simulink model "eCS_Algo_Simulation_2015b"  (R2015b)
settings: Solver=ode1  StartTime=0.0  StopTime=3  FixedStep=1/80000  RelTol=1e-3
PreLoadFcn:
  | if exist('tl_preloadfcn','file'), tl_preloadfcn(gcs,402); end
PostLoadFcn:
  | , if any(exist('dsrtsu_mdlpostloadfcn', 'file') == [2, 3, 6]), try dsrtsu_mdlpostloadfcn('Execute', bdroot); catch fprintf('Error in PostLoadFcn (dsrtsu_mdlpostloadfcn) for model "%s":\n %s\n', bdroot, lasterr); end, end,
  | if exist('tl_postloadfcn','file'), tl_postloadfcn(gcs,402); end
InitFcn:
  | Omegan=1.3024e+03;
  | xi=0.9; %0.48
  | K=0.1931;
  | K1=0.0198;
  | TauLocked=0.00255;
  | TauUnLocked=0.0042;
  | Kp=1/(2*K1);
  | Ki=Kp/((TauLocked+TauUnLocked)/2);
  | if exist('tlds_init','file'), tlds_init(gcs); end
StartFcn:
  | if exist('tlds_start','file'), tlds_start(gcs); end
StopFcn:
  | if exist('tlds_stop','file'), tlds_stop(gcs); end
model workspace (MAT data in the model file):
  au8PrevExecProfile = [0 0 0 0 0 0]
values from neighbouring files (symbols this model uses):
  AccSensor = 5    [Parameter_eCS_Algo.m]
  AlgoType = 0    [Parameter_eCS_Algo.m]
  Cxy = 1*0.017    (= 0.017)    [Acc_Init_SelV1.m]
  Cxz = 1*0.017    (= 0.017)    [Acc_Init_SelV1.m]
  Cyx = 1*0.017    (= 0.017)    [Acc_Init_SelV1.m]
  Cyz = 1*0.017    (= 0.017)    [Acc_Init_SelV1.m]
  Czx = 1*0.017    (= 0.017)    [Acc_Init_SelV1.m]
  Czy = 1*0.017    (= 0.017)    [Acc_Init_SelV1.m]
  Forced_Oscillation = 0    [Parameter_eCS_Algo.m]    (also in run_Rotation_sim.m = run)
  FreqTemperature = 10    [Acc_Init_SelV1.m]
  MaxSensorOffset = 0.3    [Acc_Init_SelV1.m]
  Mean_x_noise = 4e-3    (= 0.004)    [Acc_Init_SelV1.m]
  Mean_y_noise = 4e-3    (= 0.004)    [Acc_Init_SelV1.m]
  Mean_z_noise = 4e-3    (= 0.004)    [Acc_Init_SelV1.m]
  ODR = 8000    [Acc_Init_SelV1.m]
  offsetcorrection_on_off = 0    [Parameter_eCS_Algo.m]
  phi_pulse_rotation = 0    [Parameter_eCS_Algo.m]    (also in run_Rotation_sim.m = angle)
  pulsetype = 2    [Parameter_eCS_Algo.m]    (also in run_simulation.m = j; run_simulation_ActiveX.m = j)
  Range = 4    [Acc_Init_SelV1.m]
  sensitivity_optimisation = 0    [Parameter_eCS_Algo.m]
  TempBias = 0    [Acc_Init_SelV1.m]
  TemperatureAmp = 0    [Acc_Init_SelV1.m]
  Var_x_noise = 1.84e-9    (= 1.84e-09)    [Acc_Init_SelV1.m]
  Var_y_noise = 2.025e-09    [Acc_Init_SelV1.m]
  Var_z_noise = 1.374e-09    [Acc_Init_SelV1.m]
  w_x = 2*pi*F_x    (= 376.991118431)    [Acc_Init_SelV1.m]
  w_y = 2*pi*F_y    (= 376.991118431)    [Acc_Init_SelV1.m]
  w_z = 2*pi*F_z    (= 376.991118431)    [Acc_Init_SelV1.m]
  x_max_temp_drift = 0.061    [Acc_Init_SelV1.m]
  x_offset_enable = 0    [Acc_Init_SelV1.m]
  x_run_to_run_drift = 0.0    (= 0)    [Acc_Init_SelV1.m]
  x_temp_co_drift = 0.000    (= 0)    [Acc_Init_SelV1.m]
  Xi_x = 0.7    [Acc_Init_SelV1.m]
  Xi_y = 0.7    [Acc_Init_SelV1.m]
  Xi_z = 0.7    [Acc_Init_SelV1.m]
  y_max_temp_drift = 0.061    [Acc_Init_SelV1.m]
  y_offset_enable = 0    [Acc_Init_SelV1.m]
  y_run_to_run_drift = 0.0    (= 0)    [Acc_Init_SelV1.m]
  y_temp_co_drift = 0.000    (= 0)    [Acc_Init_SelV1.m]
  z_max_temp_drift = 0.13    [Acc_Init_SelV1.m]
  z_offset_enable = 0    [Acc_Init_SelV1.m]
  z_run_to_run_drift = 0.0    (= 0)    [Acc_Init_SelV1.m]
  z_temp_co_drift = 0.000    (= 0)    [Acc_Init_SelV1.m]
undefined symbols (not defined in the file or in its folder): controller_sample_rate, ddv, DiscIntNeverNeededParam, gmw_roada_x__m_s__, gmw_roada_y__m_s__, gmw_roadtime_2kHz, KSF_50_a_x, KSF_50_a_y, KSF_50_time, KSG_30_a_x, KSG_30_a_y, KSG_30_time, Meldorf_HindenburgstraAcceleration_x__m_s_2_, Meldorf_HindenburgstraAcceleration_y__m_s_2_, Meldorf_HindenburgstraAcceleration_z__m_s_2_, Meldorf_HindenburgstraTime__s_, pulse_FF27, pulse_MPDB, pulse_ODB40, pulse_ODB64, pulse_USNCAP, pulsetime_FF27, pulsetime_MPDB, pulsetime_ODB40, pulsetime_ODB64, pulsetime_USNCAP, Rauasphalt_60_a_x, Rauasphalt_60_a_y, Rauasphalt_60_time, sigbuilder_block, VW_416_2kHza_x_2kHz, VW_416_2kHza_y_2kHz, VW_416_2kHztime_2kHz
libraries: simulink x29, tllib x23, tl_autosar_lib x15, simulink_extras x7, LIB_TF_G_111 x2, LIB_TF_G_12_StepControl x2, LIB_TF_G_112 x1, dspsigops x1
(part 10 of 13)

== system eCS_Algo_Simulation_2015b/SAD/Subsystem/SAD/SAD/SAD_runMainFunction/SAD mainfunction/Check for following profile ==
  profile : Inport
  PrevStepIdx : Inport  Port=2
  stProfileCfg : Inport  Port=3
  Action Port : ActionPort  ActionType=then
  Check for following profile : Subsystem  TreatAsAtomicUnit=on
  Constant8 : Constant  Value=ddv('SAD/Macros/Profiles/KU8_NO_PROFILE')  mask(TL_Constant){data={'output',{'variable','SAD/Macros/Profiles/KU8_NO_PROFILE'},'date',738430.41690531245}}
      settings: CopyFcn=if exist('tl_reset_reviewflag','file')==2,tl_reset_reviewflag(gcbh);end  DeleteFcn=if exist('delete_tlblock','file')==2,delete_tlblock(gcbh);end  NameChangeFcn=if exist('rename_tlblock','file')==2,rename_tlblock(gcbh);end  OpenFcn=if exist('tl_open_blockdlg','file')==2,tl_open_blockdlg(gcbh);else,open_system(gcbh,'parameter');end
      mask Help: eval(['if exist(''tl_online_help'',''file'') == 2, tl_online_help(''Topic'',''TL_Constant''),else, web([''jar:file:///'',matlabroot,''/help/toolbox/simulink/help.jar!/slref/' lower(get_param(gcbh,'Blocktype')) '.html''], ''-helpbrowser''),end'])
      mask Display: plot([-0.1, 1.05, NaN, -0.1, 1.05],[.01, .01, NaN, .99, .99]);
  If : If  IfExpression=u1
  Keep current one : Subsystem  TreatAsAtomicUnit=on
  Merge : Merge  mask(TL_Merge){data={'date',738430.416905544}}
      settings: CopyFcn=if exist('tl_reset_reviewflag') == 2, tl_reset_reviewflag(gcbh); end  DeleteFcn=if exist('delete_tlblock','file')==2,delete_tlblock(gcbh);end  NameChangeFcn=if exist('rename_tlblock','file')==2,rename_tlblock(gcbh);end  OpenFcn=if exist('tl_open_blockdlg','file')==2,tl_open_blockdlg(gcbh);else,open_system(gcbh,'parameter');end
      mask Help: eval(['if exist(''tl_online_help'',''file'') == 2, tl_online_help(''Topic'',''TL_Merge''),else, web([''jar:file:///'',matlabroot,''/help/toolbox/simulink/help.jar!/slref/' lower(get_param(gcbh,'Blocktype')) '.html''], ''-helpbrowser''),end'])
      mask Display: plot([-0.1, 1.05, NaN, -0.1, 1.05],[.01, .01, NaN, .99, .99]);
  Relational Operator2 : RelationalOperator  Operator=~=  OutDataTypeStr=boolean  mask(TL_RelationalOperator){data={'date',738430.41690565972}}
      settings: DeleteFcn=if exist('delete_tlblock','file')==2,delete_tlblock(gcbh);end  NameChangeFcn=if exist('rename_tlblock','file')==2,rename_tlblock(gcbh);end  OpenFcn=if exist('tl_open_blockdlg','file')==2,tl_open_blockdlg(gcbh);else,open_system(gcbh,'parameter');end
      mask Help: eval(['if exist(''tl_online_help'',''file'') == 2, tl_online_help(''Topic'',''TL_RelationalOperator''),else, web([''jar:file:///'',matlabroot,''/help/toolbox/simulink/help.jar!/slref/' lower(get_param(gcbh,'Blocktype')) '.html''], ''-helpbrowser''),end'])
      mask Display: plot([-0.1, 1.05, NaN, -0.1, 1.05],[.01, .01, NaN, .99, .99]);
  selectedProfile : Outport
  wires:
  If/1 -> Check for following profile/Action
  Constant8/1 -> Relational Operator2/2
  Relational Operator2/1 -> If/1
  If/2 -> Keep current one/Action
  Check for following profile/1(Out1) -> Merge/1
  Keep current one/1(Out1) -> Merge/2
  Merge/1 -> selectedProfile/1
  PrevStepIdx/1 -> Check for following profile/1(PrevStepIdx)
  profile/1 -> Check for following profile/3(SelectedProfile), Keep current one/1(profile), Relational Operator2/1
  stProfileCfg/1 -> Check for following profile/2(stProfileCfg)

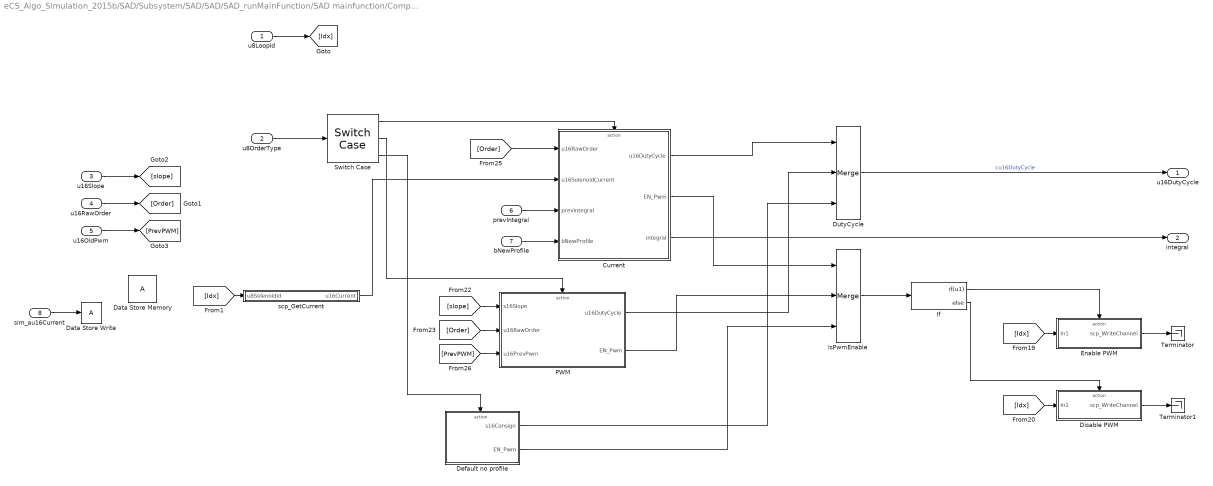
== system eCS_Algo_Simulation_2015b/SAD/Subsystem/SAD/SAD/SAD_runMainFunction/SAD mainfunction/ComputeDutyCycle ==
  u8LoopId : Inport
  u8OrderType : Inport  Port=2
  u16Slope : Inport  Port=3
  u16RawOrder : Inport  Port=4
  u16OldPwm : Inport  Port=5
  prevIntegral : Inport  Port=6
  bNewProfile : Inport  Port=7
  sim_au16Current : Inport  Port=8
  Current : Subsystem  TreatAsAtomicUnit=on
  Data Store Memory : DataStoreMemory  ReadBeforeWriteMsg=warning  WriteAfterWriteMsg=warning  WriteAfterReadMsg=warning  InitialValue=[0 0 0 0 0 0]  mask(TL_DataStoreMemory){data={'output',{'type','UInt16'},'date',738433.70621954859}}
      settings: CopyFcn=if exist('tl_reset_reviewflag') == 2, tl_reset_reviewflag(gcbh); end  DeleteFcn=if exist('delete_tlblock','file')==2,delete_tlblock(gcbh);end  NameChangeFcn=if exist('rename_tlblock','file')==2,rename_tlblock(gcbh);end  OpenFcn=if exist('tl_open_blockdlg','file')==2,tl_open_blockdlg(gcbh);else,open_system(gcbh,'parameter');end
      mask Help: eval(['if exist(''tl_online_help'',''file'') == 2, tl_online_help(''Topic'',''TL_DataStoreMemory''),else, web([''jar:file:///'',matlabroot,''/help/toolbox/simulink/help.jar!/slref/' lower(get_param(gcbh,'Blocktype')) '.html''], ''-helpbrowser''),end'])
      mask Display:
      | plot([-0.1, 1.05, NaN, -0.1, 1.05],[.01, .01, NaN, .99, .99]);
      | plot([-0.1, 1.05, NaN, -0.1, 1.05],[.01, .01, NaN, .99, .99]);
  Data Store Write : DataStoreWrite  mask(TL_DataStoreWrite){data={'date',738433.42894126161}}
      settings: DeleteFcn=if exist('delete_tlblock','file')==2,delete_tlblock(gcbh);end  NameChangeFcn=if exist('rename_tlblock','file')==2,rename_tlblock(gcbh);end  OpenFcn=if exist('tl_open_blockdlg','file')==2,tl_open_blockdlg(gcbh);else,open_system(gcbh,'parameter');end
      mask Help: eval(['if exist(''tl_online_help'',''file'') == 2, tl_online_help(''Topic'',''TL_DataStoreWrite''),else, web([''jar:file:///'',matlabroot,''/help/toolbox/simulink/help.jar!/slref/' lower(get_param(gcbh,'Blocktype')) '.html''], ''-helpbrowser''),end'])
      mask Display: plot([-0.1, 1.05, NaN, -0.1, 1.05],[.01, .01, NaN, .99, .99]);
  Default no profile : Subsystem  TreatAsAtomicUnit=on
  Disable PWM : Subsystem  TreatAsAtomicUnit=on
  DutyCycle : Merge  Inputs=3  mask(TL_Merge){data={'date',738430.41690787033}}
      settings: CopyFcn=if exist('tl_reset_reviewflag') == 2, tl_reset_reviewflag(gcbh); end  DeleteFcn=if exist('delete_tlblock','file')==2,delete_tlblock(gcbh);end  NameChangeFcn=if exist('rename_tlblock','file')==2,rename_tlblock(gcbh);end  OpenFcn=if exist('tl_open_blockdlg','file')==2,tl_open_blockdlg(gcbh);else,open_system(gcbh,'parameter');end
      mask Help: eval(['if exist(''tl_online_help'',''file'') == 2, tl_online_help(''Topic'',''TL_Merge''),else, web([''jar:file:///'',matlabroot,''/help/toolbox/simulink/help.jar!/slref/' lower(get_param(gcbh,'Blocktype')) '.html''], ''-helpbrowser''),end'])
      mask Display: plot([-0.1, 1.05, NaN, -0.1, 1.05],[.01, .01, NaN, .99, .99]);
  Enable PWM : Subsystem  TreatAsAtomicUnit=on
  If : If  IfExpression=u1
  IsPwmEnable : Merge  Inputs=3  mask(TL_Merge){data={'date',738430.41690775461}}
      settings: CopyFcn=if exist('tl_reset_reviewflag') == 2, tl_reset_reviewflag(gcbh); end  DeleteFcn=if exist('delete_tlblock','file')==2,delete_tlblock(gcbh);end  NameChangeFcn=if exist('rename_tlblock','file')==2,rename_tlblock(gcbh);end  OpenFcn=if exist('tl_open_blockdlg','file')==2,tl_open_blockdlg(gcbh);else,open_system(gcbh,'parameter');end
      mask Help: eval(['if exist(''tl_online_help'',''file'') == 2, tl_online_help(''Topic'',''TL_Merge''),else, web([''jar:file:///'',matlabroot,''/help/toolbox/simulink/help.jar!/slref/' lower(get_param(gcbh,'Blocktype')) '.html''], ''-helpbrowser''),end'])
      mask Display: plot([-0.1, 1.05, NaN, -0.1, 1.05],[.01, .01, NaN, .99, .99]);
  PWM : Subsystem  TreatAsAtomicUnit=on
  Switch Case : SwitchCase  CaseConditions={1,2}
  Terminator : Terminator
  Terminator1 : Terminator
  scp_GetCurrent : Subsystem  TreatAsAtomicUnit=on
  u16DutyCycle : Outport
  integral : Outport  Port=2
  wires:
  u8OrderType/1 -> Switch Case/1
  Switch Case/3 -> Default no profile/Action
  Default no profile/2(EN_Pwm) -> IsPwmEnable/3
  If/1 -> Enable PWM/Action
  Default no profile/1(s16Consign) -> DutyCycle/3
  [Idx] -> Disable PWM/1(In1)
  Disable PWM/1(scp_WriteChannel) -> Terminator1/1
  [PrevPWM] -> PWM/3(u16PrevPwm)
  [Order] -> Current/1(u16RawOrder)
  [Order] -> PWM/2(u16RawOrder)
  Enable PWM/1(scp_WriteChannel) -> Terminator/1
  [Idx] -> Enable PWM/1(In1)
  If/2 -> Disable PWM/Action
  [slope] -> PWM/1(s16Slope)
  DutyCycle/1 -> u16DutyCycle/1  "cu16DutyCycle"
  Switch Case/1 -> Current/Action
  Switch Case/2 -> PWM/Action
  u8LoopId/1 -> [Idx]
  u16RawOrder/1 -> [Order]
  u16Slope/1 -> [slope]
  u16OldPwm/1 -> [PrevPWM]
  IsPwmEnable/1 -> If/1
  [Idx] -> scp_GetCurrent/1(u8SolenoidId)
  scp_GetCurrent/1(u16Current) -> Current/2(u16SolenoidCurrent)
  Current/3(integral) -> integral/1
  prevIntegral/1 -> Current/3(prevIntegral)
  bNewProfile/1 -> Current/4(bNewProfile)
  sim_au16Current/1 -> Data Store Write/1
  Current/2(EN_Pwm) -> IsPwmEnable/1
  PWM/2(EN_Pwm) -> IsPwmEnable/2
  Current/1(u16DutyCycle) -> DutyCycle/1
  PWM/1(u16DutyCycle) -> DutyCycle/2

== system eCS_Algo_Simulation_2015b/SAD/Subsystem/SAD/SAD/SAD_runMainFunction/SAD mainfunction/Keep current profile ==
  PrevProfile : Inport
  Action Port : ActionPort  ActionType=else
  SelectedProfile : Outport
  wires:
  PrevProfile/1 -> SelectedProfile/1

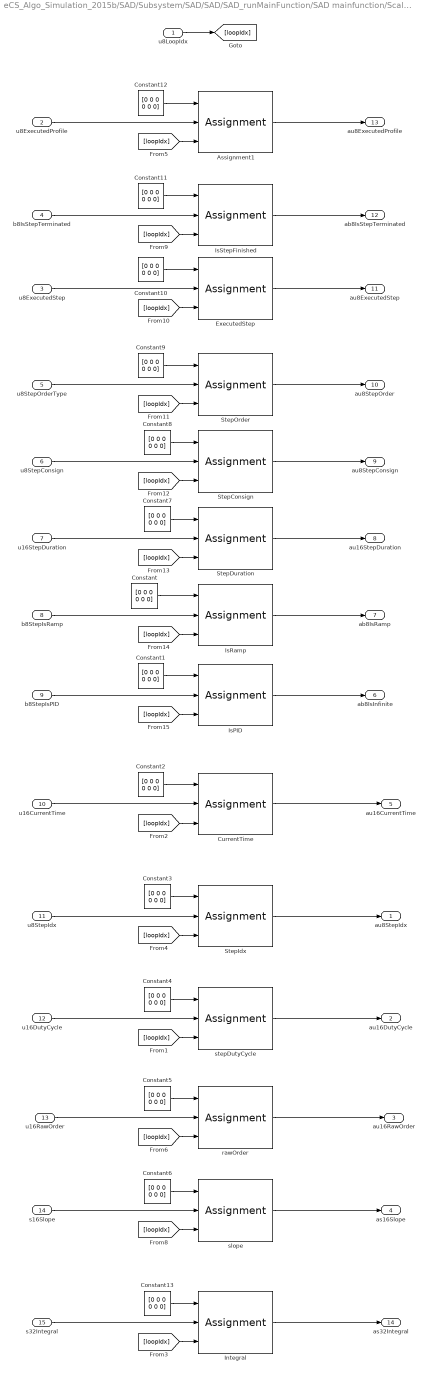
== system eCS_Algo_Simulation_2015b/SAD/Subsystem/SAD/SAD/SAD_runMainFunction/SAD mainfunction/ScalarToVector ==
  u8LoopIdx : Inport
  u8ExecutedProfile : Inport  Port=2
  u8ExecutedStep : Inport  Port=3
  b8IsStepTerminated : Inport  Port=4
  u8StepOrderType : Inport  Port=5
  u8StepConsign : Inport  Port=6
  u16StepDuration : Inport  Port=7
  b8StepIsRamp : Inport  Port=8
  b8StepIsPID : Inport  Port=9
  u16CurrentTime : Inport  Port=10
  u8StepIdx : Inport  Port=11
  u16DutyCycle : Inport  Port=12
  u16RawOrder : Inport  Port=13
  s16Slope : Inport  Port=14
  s32Integral : Inport  Port=15
  Assignment1 : Assignment  IndexMode=Zero-based  IndexOptions=Index vector (port)  Indices=1  OutputSizes=1  mask(TL_Assignment){data={'insideiteratedsystem',logical(1),'omitinitializations',1,'output',{'variable','SAD/Vars/Profiles/au8ExecProfile','inheritscaling',0},'date',738430.41691026615}}
      settings: CopyFcn=if exist('tl_reset_reviewflag') == 2, tl_reset_reviewflag(gcbh); end  DeleteFcn=if exist('delete_tlblock','file')==2,delete_tlblock(gcbh);end  NameChangeFcn=if exist('rename_tlblock','file')==2,rename_tlblock(gcbh);end  OpenFcn=if exist('tl_open_blockdlg','file')==2,tl_open_blockdlg(gcbh);else,open_system(gcbh,'parameter');end
      mask Help: eval(['if exist(''tl_online_help'',''file'') == 2, tl_online_help(''Topic'',''TL_Assignment''),else, web([''jar:file:///'',matlabroot,''/help/toolbox/simulink/help.jar!/slref/' lower(get_param(gcbh,'Blocktype')) '.html''], ''-helpbrowser''),end'])
      mask Display: plot([-0.1, 1.05, NaN, -0.1, 1.05],[.01, .01, NaN, .99, .99]);
  Constant : Constant  Value=[0 0 0 0 0 0]  mask(TL_Constant){data={'date',738430.41691038199}}
      settings: CopyFcn=if exist('tl_reset_reviewflag') == 2, tl_reset_reviewflag(gcbh); end  DeleteFcn=if exist('delete_tlblock','file')==2,delete_tlblock(gcbh);end  NameChangeFcn=if exist('rename_tlblock','file')==2,rename_tlblock(gcbh);end  OpenFcn=if exist('tl_open_blockdlg','file')==2,tl_open_blockdlg(gcbh);else,open_system(gcbh,'parameter');end
      mask Help: eval(['if exist(''tl_online_help'',''file'') == 2, tl_online_help(''Topic'',''TL_Constant''),else, web([''jar:file:///'',matlabroot,''/help/toolbox/simulink/help.jar!/slref/' lower(get_param(gcbh,'Blocktype')) '.html''], ''-helpbrowser''),end'])
      mask Display: plot([-0.1, 1.05, NaN, -0.1, 1.05],[.01, .01, NaN, .99, .99]);
  Constant1 : Constant  Value=[0 0 0 0 0 0]  mask(TL_Constant){data={'date',738430.4169104977}}
      settings: CopyFcn=if exist('tl_reset_reviewflag') == 2, tl_reset_reviewflag(gcbh); end  DeleteFcn=if exist('delete_tlblock','file')==2,delete_tlblock(gcbh);end  NameChangeFcn=if exist('rename_tlblock','file')==2,rename_tlblock(gcbh);end  OpenFcn=if exist('tl_open_blockdlg','file')==2,tl_open_blockdlg(gcbh);else,open_system(gcbh,'parameter');end
      mask Help: eval(['if exist(''tl_online_help'',''file'') == 2, tl_online_help(''Topic'',''TL_Constant''),else, web([''jar:file:///'',matlabroot,''/help/toolbox/simulink/help.jar!/slref/' lower(get_param(gcbh,'Blocktype')) '.html''], ''-helpbrowser''),end'])
      mask Display: plot([-0.1, 1.05, NaN, -0.1, 1.05],[.01, .01, NaN, .99, .99]);
  Constant10 : Constant  Value=[0 0 0 0 0 0]  mask(TL_Constant){data={'date',738430.41691072914}}
      settings: CopyFcn=if exist('tl_reset_reviewflag') == 2, tl_reset_reviewflag(gcbh); end  DeleteFcn=if exist('delete_tlblock','file')==2,delete_tlblock(gcbh);end  NameChangeFcn=if exist('rename_tlblock','file')==2,rename_tlblock(gcbh);end  OpenFcn=if exist('tl_open_blockdlg','file')==2,tl_open_blockdlg(gcbh);else,open_system(gcbh,'parameter');end
      mask Help: eval(['if exist(''tl_online_help'',''file'') == 2, tl_online_help(''Topic'',''TL_Constant''),else, web([''jar:file:///'',matlabroot,''/help/toolbox/simulink/help.jar!/slref/' lower(get_param(gcbh,'Blocktype')) '.html''], ''-helpbrowser''),end'])
      mask Display: plot([-0.1, 1.05, NaN, -0.1, 1.05],[.01, .01, NaN, .99, .99]);
  Constant11 : Constant  Value=[0 0 0 0 0 0]  mask(TL_Constant){data={'date',738430.4169108565}}
      settings: CopyFcn=if exist('tl_reset_reviewflag') == 2, tl_reset_reviewflag(gcbh); end  DeleteFcn=if exist('delete_tlblock','file')==2,delete_tlblock(gcbh);end  NameChangeFcn=if exist('rename_tlblock','file')==2,rename_tlblock(gcbh);end  OpenFcn=if exist('tl_open_blockdlg','file')==2,tl_open_blockdlg(gcbh);else,open_system(gcbh,'parameter');end
      mask Help: eval(['if exist(''tl_online_help'',''file'') == 2, tl_online_help(''Topic'',''TL_Constant''),else, web([''jar:file:///'',matlabroot,''/help/toolbox/simulink/help.jar!/slref/' lower(get_param(gcbh,'Blocktype')) '.html''], ''-helpbrowser''),end'])
      mask Display: plot([-0.1, 1.05, NaN, -0.1, 1.05],[.01, .01, NaN, .99, .99]);
  Constant12 : Constant  Value=[0 0 0 0 0 0]  mask(TL_Constant){data={'date',738430.41691097221}}
      settings: CopyFcn=if exist('tl_reset_reviewflag') == 2, tl_reset_reviewflag(gcbh); end  DeleteFcn=if exist('delete_tlblock','file')==2,delete_tlblock(gcbh);end  NameChangeFcn=if exist('rename_tlblock','file')==2,rename_tlblock(gcbh);end  OpenFcn=if exist('tl_open_blockdlg','file')==2,tl_open_blockdlg(gcbh);else,open_system(gcbh,'parameter');end
      mask Help: eval(['if exist(''tl_online_help'',''file'') == 2, tl_online_help(''Topic'',''TL_Constant''),else, web([''jar:file:///'',matlabroot,''/help/toolbox/simulink/help.jar!/slref/' lower(get_param(gcbh,'Blocktype')) '.html''], ''-helpbrowser''),end'])
      mask Display: plot([-0.1, 1.05, NaN, -0.1, 1.05],[.01, .01, NaN, .99, .99]);
  Constant13 : Constant  Value=[0 0 0 0 0 0]  mask(TL_Constant){data={'date',738430.41691166663}}
      settings: CopyFcn=if exist('tl_reset_reviewflag') == 2, tl_reset_reviewflag(gcbh); end  DeleteFcn=if exist('delete_tlblock','file')==2,delete_tlblock(gcbh);end  NameChangeFcn=if exist('rename_tlblock','file')==2,rename_tlblock(gcbh);end  OpenFcn=if exist('tl_open_blockdlg','file')==2,tl_open_blockdlg(gcbh);else,open_system(gcbh,'parameter');end
      mask Help: eval(['if exist(''tl_online_help'',''file'') == 2, tl_online_help(''Topic'',''TL_Constant''),else, web([''jar:file:///'',matlabroot,''/help/toolbox/simulink/help.jar!/slref/' lower(get_param(gcbh,'Blocktype')) '.html''], ''-helpbrowser''),end'])
      mask Display: plot([-0.1, 1.05, NaN, -0.1, 1.05],[.01, .01, NaN, .99, .99]);
  Constant2 : Constant  Value=[0 0 0 0 0 0]  mask(TL_Constant){data={'date',738430.41691108793}}
      settings: CopyFcn=if exist('tl_reset_reviewflag') == 2, tl_reset_reviewflag(gcbh); end  DeleteFcn=if exist('delete_tlblock','file')==2,delete_tlblock(gcbh);end  NameChangeFcn=if exist('rename_tlblock','file')==2,rename_tlblock(gcbh);end  OpenFcn=if exist('tl_open_blockdlg','file')==2,tl_open_blockdlg(gcbh);else,open_system(gcbh,'parameter');end
      mask Help: eval(['if exist(''tl_online_help'',''file'') == 2, tl_online_help(''Topic'',''TL_Constant''),else, web([''jar:file:///'',matlabroot,''/help/toolbox/simulink/help.jar!/slref/' lower(get_param(gcbh,'Blocktype')) '.html''], ''-helpbrowser''),end'])
      mask Display: plot([-0.1, 1.05, NaN, -0.1, 1.05],[.01, .01, NaN, .99, .99]);
  Constant3 : Constant  Value=[0 0 0 0 0 0]  mask(TL_Constant){data={'date',738430.41691120365}}
      settings: CopyFcn=if exist('tl_reset_reviewflag') == 2, tl_reset_reviewflag(gcbh); end  DeleteFcn=if exist('delete_tlblock','file')==2,delete_tlblock(gcbh);end  NameChangeFcn=if exist('rename_tlblock','file')==2,rename_tlblock(gcbh);end  OpenFcn=if exist('tl_open_blockdlg','file')==2,tl_open_blockdlg(gcbh);else,open_system(gcbh,'parameter');end
      mask Help: eval(['if exist(''tl_online_help'',''file'') == 2, tl_online_help(''Topic'',''TL_Constant''),else, web([''jar:file:///'',matlabroot,''/help/toolbox/simulink/help.jar!/slref/' lower(get_param(gcbh,'Blocktype')) '.html''], ''-helpbrowser''),end'])
      mask Display: plot([-0.1, 1.05, NaN, -0.1, 1.05],[.01, .01, NaN, .99, .99]);
  Constant4 : Constant  Value=[0 0 0 0 0 0]  mask(TL_Constant){data={'date',738430.41691131948}}
      settings: CopyFcn=if exist('tl_reset_reviewflag') == 2, tl_reset_reviewflag(gcbh); end  DeleteFcn=if exist('delete_tlblock','file')==2,delete_tlblock(gcbh);end  NameChangeFcn=if exist('rename_tlblock','file')==2,rename_tlblock(gcbh);end  OpenFcn=if exist('tl_open_blockdlg','file')==2,tl_open_blockdlg(gcbh);else,open_system(gcbh,'parameter');end
      mask Help: eval(['if exist(''tl_online_help'',''file'') == 2, tl_online_help(''Topic'',''TL_Constant''),else, web([''jar:file:///'',matlabroot,''/help/toolbox/simulink/help.jar!/slref/' lower(get_param(gcbh,'Blocktype')) '.html''], ''-helpbrowser''),end'])
      mask Display: plot([-0.1, 1.05, NaN, -0.1, 1.05],[.01, .01, NaN, .99, .99]);
  Constant5 : Constant  Value=[0 0 0 0 0 0]  mask(TL_Constant){data={'date',738430.41691155091}}
      settings: CopyFcn=if exist('tl_reset_reviewflag') == 2, tl_reset_reviewflag(gcbh); end  DeleteFcn=if exist('delete_tlblock','file')==2,delete_tlblock(gcbh);end  NameChangeFcn=if exist('rename_tlblock','file')==2,rename_tlblock(gcbh);end  OpenFcn=if exist('tl_open_blockdlg','file')==2,tl_open_blockdlg(gcbh);else,open_system(gcbh,'parameter');end
      mask Help: eval(['if exist(''tl_online_help'',''file'') == 2, tl_online_help(''Topic'',''TL_Constant''),else, web([''jar:file:///'',matlabroot,''/help/toolbox/simulink/help.jar!/slref/' lower(get_param(gcbh,'Blocktype')) '.html''], ''-helpbrowser''),end'])
      mask Display: plot([-0.1, 1.05, NaN, -0.1, 1.05],[.01, .01, NaN, .99, .99]);
  Constant6 : Constant  Value=[0 0 0 0 0 0]  mask(TL_Constant){data={'date',738430.41691166663}}
      settings: CopyFcn=if exist('tl_reset_reviewflag') == 2, tl_reset_reviewflag(gcbh); end  DeleteFcn=if exist('delete_tlblock','file')==2,delete_tlblock(gcbh);end  NameChangeFcn=if exist('rename_tlblock','file')==2,rename_tlblock(gcbh);end  OpenFcn=if exist('tl_open_blockdlg','file')==2,tl_open_blockdlg(gcbh);else,open_system(gcbh,'parameter');end
      mask Help: eval(['if exist(''tl_online_help'',''file'') == 2, tl_online_help(''Topic'',''TL_Constant''),else, web([''jar:file:///'',matlabroot,''/help/toolbox/simulink/help.jar!/slref/' lower(get_param(gcbh,'Blocktype')) '.html''], ''-helpbrowser''),end'])
      mask Display: plot([-0.1, 1.05, NaN, -0.1, 1.05],[.01, .01, NaN, .99, .99]);
  Constant7 : Constant  Value=[0 0 0 0 0 0]  mask(TL_Constant){data={'date',738430.41691178246}}
      settings: CopyFcn=if exist('tl_reset_reviewflag') == 2, tl_reset_reviewflag(gcbh); end  DeleteFcn=if exist('delete_tlblock','file')==2,delete_tlblock(gcbh);end  NameChangeFcn=if exist('rename_tlblock','file')==2,rename_tlblock(gcbh);end  OpenFcn=if exist('tl_open_blockdlg','file')==2,tl_open_blockdlg(gcbh);else,open_system(gcbh,'parameter');end
      mask Help: eval(['if exist(''tl_online_help'',''file'') == 2, tl_online_help(''Topic'',''TL_Constant''),else, web([''jar:file:///'',matlabroot,''/help/toolbox/simulink/help.jar!/slref/' lower(get_param(gcbh,'Blocktype')) '.html''], ''-helpbrowser''),end'])
      mask Display: plot([-0.1, 1.05, NaN, -0.1, 1.05],[.01, .01, NaN, .99, .99]);
  Constant8 : Constant  Value=[0 0 0 0 0 0]  mask(TL_Constant){data={'date',738430.41691189818}}
      settings: CopyFcn=if exist('tl_reset_reviewflag') == 2, tl_reset_reviewflag(gcbh); end  DeleteFcn=if exist('delete_tlblock','file')==2,delete_tlblock(gcbh);end  NameChangeFcn=if exist('rename_tlblock','file')==2,rename_tlblock(gcbh);end  OpenFcn=if exist('tl_open_blockdlg','file')==2,tl_open_blockdlg(gcbh);else,open_system(gcbh,'parameter');end
      mask Help: eval(['if exist(''tl_online_help'',''file'') == 2, tl_online_help(''Topic'',''TL_Constant''),else, web([''jar:file:///'',matlabroot,''/help/toolbox/simulink/help.jar!/slref/' lower(get_param(gcbh,'Blocktype')) '.html''], ''-helpbrowser''),end'])
      mask Display: plot([-0.1, 1.05, NaN, -0.1, 1.05],[.01, .01, NaN, .99, .99]);
  Constant9 : Constant  Value=[0 0 0 0 0 0]  mask(TL_Constant){data={'date',738430.41691199073}}
      settings: CopyFcn=if exist('tl_reset_reviewflag') == 2, tl_reset_reviewflag(gcbh); end  DeleteFcn=if exist('delete_tlblock','file')==2,delete_tlblock(gcbh);end  NameChangeFcn=if exist('rename_tlblock','file')==2,rename_tlblock(gcbh);end  OpenFcn=if exist('tl_open_blockdlg','file')==2,tl_open_blockdlg(gcbh);else,open_system(gcbh,'parameter');end
      mask Help: eval(['if exist(''tl_online_help'',''file'') == 2, tl_online_help(''Topic'',''TL_Constant''),else, web([''jar:file:///'',matlabroot,''/help/toolbox/simulink/help.jar!/slref/' lower(get_param(gcbh,'Blocktype')) '.html''], ''-helpbrowser''),end'])
      mask Display: plot([-0.1, 1.05, NaN, -0.1, 1.05],[.01, .01, NaN, .99, .99]);
  CurrentTime : Assignment  IndexMode=Zero-based  IndexOptions=Index vector (port)  Indices=1  OutputSizes=1  mask(TL_Assignment){data={'insideiteratedsystem',logical(1),'omitinitializations',1,'output',{'variable','SAD/Vars/Steps/au16Time','inheritscaling',0},'date',738430.41691224533}}
      settings: CopyFcn=if exist('tl_reset_reviewflag') == 2, tl_reset_reviewflag(gcbh); end  DeleteFcn=if exist('delete_tlblock','file')==2,delete_tlblock(gcbh);end  NameChangeFcn=if exist('rename_tlblock','file')==2,rename_tlblock(gcbh);end  OpenFcn=if exist('tl_open_blockdlg','file')==2,tl_open_blockdlg(gcbh);else,open_system(gcbh,'parameter');end
      mask Help: eval(['if exist(''tl_online_help'',''file'') == 2, tl_online_help(''Topic'',''TL_Assignment''),else, web([''jar:file:///'',matlabroot,''/help/toolbox/simulink/help.jar!/slref/' lower(get_param(gcbh,'Blocktype')) '.html''], ''-helpbrowser''),end'])
      mask Display: plot([-0.1, 1.05, NaN, -0.1, 1.05],[.01, .01, NaN, .99, .99]);
  ExecutedStep : Assignment  IndexMode=Zero-based  IndexOptions=Index vector (port)  Indices=1  OutputSizes=1  mask(TL_Assignment){data={'insideiteratedsystem',logical(1),'omitinitializations',1,'output',{'variable','SAD/Vars/Steps/au8ExecutedStep','inheritscaling',0},'date',738430.41691236116}}
      settings: CopyFcn=if exist('tl_reset_reviewflag') == 2, tl_reset_reviewflag(gcbh); end  DeleteFcn=if exist('delete_tlblock','file')==2,delete_tlblock(gcbh);end  NameChangeFcn=if exist('rename_tlblock','file')==2,rename_tlblock(gcbh);end  OpenFcn=if exist('tl_open_blockdlg','file')==2,tl_open_blockdlg(gcbh);else,open_system(gcbh,'parameter');end
      mask Help: eval(['if exist(''tl_online_help'',''file'') == 2, tl_online_help(''Topic'',''TL_Assignment''),else, web([''jar:file:///'',matlabroot,''/help/toolbox/simulink/help.jar!/slref/' lower(get_param(gcbh,'Blocktype')) '.html''], ''-helpbrowser''),end'])
      mask Display: plot([-0.1, 1.05, NaN, -0.1, 1.05],[.01, .01, NaN, .99, .99]);
  Integral : Assignment  IndexMode=Zero-based  IndexOptions=Index vector (port)  Indices=1  OutputSizes=1  mask(TL_Assignment){data={'insideiteratedsystem',logical(1),'omitinitializations',1,'output',{'variable','SAD/Vars/Steps/as32Integral','inheritscaling',0},'date',738430.55898019671}}
      settings: CopyFcn=if exist('tl_reset_reviewflag') == 2, tl_reset_reviewflag(gcbh); end  DeleteFcn=if exist('delete_tlblock','file')==2,delete_tlblock(gcbh);end  NameChangeFcn=if exist('rename_tlblock','file')==2,rename_tlblock(gcbh);end  OpenFcn=if exist('tl_open_blockdlg','file')==2,tl_open_blockdlg(gcbh);else,open_system(gcbh,'parameter');end
      mask Help: eval(['if exist(''tl_online_help'',''file'') == 2, tl_online_help(''Topic'',''TL_Assignment''),else, web([''jar:file:///'',matlabroot,''/help/toolbox/simulink/help.jar!/slref/' lower(get_param(gcbh,'Blocktype')) '.html''], ''-helpbrowser''),end'])
      mask Display: plot([-0.1, 1.05, NaN, -0.1, 1.05],[.01, .01, NaN, .99, .99]);
  IsPID : Assignment  IndexMode=Zero-based  IndexOptions=Index vector (port)  Indices=1  OutputSizes=1  mask(TL_Assignment){data={'insideiteratedsystem',logical(1),'omitinitializations',1,'output',{'variable','SAD/Vars/Steps/astSteps/Components/ab8IsPID','inheritscaling',0},'date',738430.41691270832}}
      settings: CopyFcn=if exist('tl_reset_reviewflag') == 2, tl_reset_reviewflag(gcbh); end  DeleteFcn=if exist('delete_tlblock','file')==2,delete_tlblock(gcbh);end  NameChangeFcn=if exist('rename_tlblock','file')==2,rename_tlblock(gcbh);end  OpenFcn=if exist('tl_open_blockdlg','file')==2,tl_open_blockdlg(gcbh);else,open_system(gcbh,'parameter');end
      mask Help: eval(['if exist(''tl_online_help'',''file'') == 2, tl_online_help(''Topic'',''TL_Assignment''),else, web([''jar:file:///'',matlabroot,''/help/toolbox/simulink/help.jar!/slref/' lower(get_param(gcbh,'Blocktype')) '.html''], ''-helpbrowser''),end'])
      mask Display: plot([-0.1, 1.05, NaN, -0.1, 1.05],[.01, .01, NaN, .99, .99]);
  IsRamp : Assignment  IndexMode=Zero-based  IndexOptions=Index vector (port)  Indices=1  OutputSizes=1  mask(TL_Assignment){data={'insideiteratedsystem',logical(1),'omitinitializations',1,'output',{'variable','SAD/Vars/Steps/astSteps/Components/ab8IsRamp','inheritscaling',0},'date',738430.41691293987}}
      settings: CopyFcn=if exist('tl_reset_reviewflag') == 2, tl_reset_reviewflag(gcbh); end  DeleteFcn=if exist('delete_tlblock','file')==2,delete_tlblock(gcbh);end  NameChangeFcn=if exist('rename_tlblock','file')==2,rename_tlblock(gcbh);end  OpenFcn=if exist('tl_open_blockdlg','file')==2,tl_open_blockdlg(gcbh);else,open_system(gcbh,'parameter');end
      mask Help: eval(['if exist(''tl_online_help'',''file'') == 2, tl_online_help(''Topic'',''TL_Assignment''),else, web([''jar:file:///'',matlabroot,''/help/toolbox/simulink/help.jar!/slref/' lower(get_param(gcbh,'Blocktype')) '.html''], ''-helpbrowser''),end'])
      mask Display: plot([-0.1, 1.05, NaN, -0.1, 1.05],[.01, .01, NaN, .99, .99]);
  IsStepFinished : Assignment  IndexMode=Zero-based  IndexOptions=Index vector (port)  Indices=1  OutputSizes=1  mask(TL_Assignment){data={'insideiteratedsystem',logical(1),'omitinitializations',1,'output',{'variable','SAD/Vars/Steps/ab8IsStepFinished','inheritscaling',0},'date',738430.41691305558}}
      settings: CopyFcn=if exist('tl_reset_reviewflag') == 2, tl_reset_reviewflag(gcbh); end  DeleteFcn=if exist('delete_tlblock','file')==2,delete_tlblock(gcbh);end  NameChangeFcn=if exist('rename_tlblock','file')==2,rename_tlblock(gcbh);end  OpenFcn=if exist('tl_open_blockdlg','file')==2,tl_open_blockdlg(gcbh);else,open_system(gcbh,'parameter');end
      mask Help: eval(['if exist(''tl_online_help'',''file'') == 2, tl_online_help(''Topic'',''TL_Assignment''),else, web([''jar:file:///'',matlabroot,''/help/toolbox/simulink/help.jar!/slref/' lower(get_param(gcbh,'Blocktype')) '.html''], ''-helpbrowser''),end'])
      mask Display: plot([-0.1, 1.05, NaN, -0.1, 1.05],[.01, .01, NaN, .99, .99]);
  StepConsign : Assignment  IndexMode=Zero-based  IndexOptions=Index vector (port)  Indices=1  OutputSizes=1  mask(TL_Assignment){data={'insideiteratedsystem',logical(1),'omitinitializations',1,'output',{'variable','SAD/Vars/Steps/astSteps/Components/au8Consign','inheritscaling',0},'date',738430.41691327549}}
      settings: CopyFcn=if exist('tl_reset_reviewflag') == 2, tl_reset_reviewflag(gcbh); end  DeleteFcn=if exist('delete_tlblock','file')==2,delete_tlblock(gcbh);end  NameChangeFcn=if exist('rename_tlblock','file')==2,rename_tlblock(gcbh);end  OpenFcn=if exist('tl_open_blockdlg','file')==2,tl_open_blockdlg(gcbh);else,open_system(gcbh,'parameter');end
      mask Help: eval(['if exist(''tl_online_help'',''file'') == 2, tl_online_help(''Topic'',''TL_Assignment''),else, web([''jar:file:///'',matlabroot,''/help/toolbox/simulink/help.jar!/slref/' lower(get_param(gcbh,'Blocktype')) '.html''], ''-helpbrowser''),end'])
      mask Display: plot([-0.1, 1.05, NaN, -0.1, 1.05],[.01, .01, NaN, .99, .99]);
  StepDuration : Assignment  IndexMode=Zero-based  IndexOptions=Index vector (port)  Indices=1  OutputSizes=1  mask(TL_Assignment){data={'insideiteratedsystem',logical(1),'omitinitializations',1,'output',{'variable','SAD/Vars/Steps/astSteps/Components/au16Duration','inheritscaling',0},'date',738430.41691339121}}
      settings: CopyFcn=if exist('tl_reset_reviewflag') == 2, tl_reset_reviewflag(gcbh); end  DeleteFcn=if exist('delete_tlblock','file')==2,delete_tlblock(gcbh);end  NameChangeFcn=if exist('rename_tlblock','file')==2,rename_tlblock(gcbh);end  OpenFcn=if exist('tl_open_blockdlg','file')==2,tl_open_blockdlg(gcbh);else,open_system(gcbh,'parameter');end
      mask Help: eval(['if exist(''tl_online_help'',''file'') == 2, tl_online_help(''Topic'',''TL_Assignment''),else, web([''jar:file:///'',matlabroot,''/help/toolbox/simulink/help.jar!/slref/' lower(get_param(gcbh,'Blocktype')) '.html''], ''-helpbrowser''),end'])
      mask Display: plot([-0.1, 1.05, NaN, -0.1, 1.05],[.01, .01, NaN, .99, .99]);
  StepIdx : Assignment  IndexMode=Zero-based  IndexOptions=Index vector (port)  Indices=1  OutputSizes=1  mask(TL_Assignment){data={'insideiteratedsystem',logical(1),'omitinitializations',1,'output',{'variable','SAD/Vars/Steps/au8StepIdx','inheritscaling',0},'date',738430.41691363428}}
      settings: CopyFcn=if exist('tl_reset_reviewflag') == 2, tl_reset_reviewflag(gcbh); end  DeleteFcn=if exist('delete_tlblock','file')==2,delete_tlblock(gcbh);end  NameChangeFcn=if exist('rename_tlblock','file')==2,rename_tlblock(gcbh);end  OpenFcn=if exist('tl_open_blockdlg','file')==2,tl_open_blockdlg(gcbh);else,open_system(gcbh,'parameter');end
      mask Help: eval(['if exist(''tl_online_help'',''file'') == 2, tl_online_help(''Topic'',''TL_Assignment''),else, web([''jar:file:///'',matlabroot,''/help/toolbox/simulink/help.jar!/slref/' lower(get_param(gcbh,'Blocktype')) '.html''], ''-helpbrowser''),end'])
      mask Display: plot([-0.1, 1.05, NaN, -0.1, 1.05],[.01, .01, NaN, .99, .99]);
  StepOrder : Assignment  IndexMode=Zero-based  IndexOptions=Index vector (port)  Indices=1  OutputSizes=1  mask(TL_Assignment){data={'insideiteratedsystem',logical(1),'omitinitializations',1,'output',{'variable','SAD/Vars/Steps/astSteps/Components/au8OrderType','inheritscaling',0},'date',738430.41691375}}
      settings: CopyFcn=if exist('tl_reset_reviewflag') == 2, tl_reset_reviewflag(gcbh); end  DeleteFcn=if exist('delete_tlblock','file')==2,delete_tlblock(gcbh);end  NameChangeFcn=if exist('rename_tlblock','file')==2,rename_tlblock(gcbh);end  OpenFcn=if exist('tl_open_blockdlg','file')==2,tl_open_blockdlg(gcbh);else,open_system(gcbh,'parameter');end
      mask Help: eval(['if exist(''tl_online_help'',''file'') == 2, tl_online_help(''Topic'',''TL_Assignment''),else, web([''jar:file:///'',matlabroot,''/help/toolbox/simulink/help.jar!/slref/' lower(get_param(gcbh,'Blocktype')) '.html''], ''-helpbrowser''),end'])
      mask Display: plot([-0.1, 1.05, NaN, -0.1, 1.05],[.01, .01, NaN, .99, .99]);
  rawOrder : Assignment  IndexMode=Zero-based  IndexOptions=Index vector (port)  Indices=1  OutputSizes=1  mask(TL_Assignment){data={'insideiteratedsystem',logical(1),'omitinitializations',1,'output',{'variable','SAD/Vars/Steps/au16RawOrder','inheritscaling',0},'date',738430.41691398143}}
      settings: CopyFcn=if exist('tl_reset_reviewflag') == 2, tl_reset_reviewflag(gcbh); end  DeleteFcn=if exist('delete_tlblock','file')==2,delete_tlblock(gcbh);end  NameChangeFcn=if exist('rename_tlblock','file')==2,rename_tlblock(gcbh);end  OpenFcn=if exist('tl_open_blockdlg','file')==2,tl_open_blockdlg(gcbh);else,open_system(gcbh,'parameter');end
      mask Help: eval(['if exist(''tl_online_help'',''file'') == 2, tl_online_help(''Topic'',''TL_Assignment''),else, web([''jar:file:///'',matlabroot,''/help/toolbox/simulink/help.jar!/slref/' lower(get_param(gcbh,'Blocktype')) '.html''], ''-helpbrowser''),end'])
      mask Display: plot([-0.1, 1.05, NaN, -0.1, 1.05],[.01, .01, NaN, .99, .99]);
  slope : Assignment  IndexMode=Zero-based  IndexOptions=Index vector (port)  Indices=1  OutputSizes=1  mask(TL_Assignment){data={'insideiteratedsystem',logical(1),'omitinitializations',1,'output',{'variable','SAD/Vars/Steps/as16Slope','inheritscaling',0},'date',738430.41691409727}}
      settings: CopyFcn=if exist('tl_reset_reviewflag') == 2, tl_reset_reviewflag(gcbh); end  DeleteFcn=if exist('delete_tlblock','file')==2,delete_tlblock(gcbh);end  NameChangeFcn=if exist('rename_tlblock','file')==2,rename_tlblock(gcbh);end  OpenFcn=if exist('tl_open_blockdlg','file')==2,tl_open_blockdlg(gcbh);else,open_system(gcbh,'parameter');end
      mask Help: eval(['if exist(''tl_online_help'',''file'') == 2, tl_online_help(''Topic'',''TL_Assignment''),else, web([''jar:file:///'',matlabroot,''/help/toolbox/simulink/help.jar!/slref/' lower(get_param(gcbh,'Blocktype')) '.html''], ''-helpbrowser''),end'])
      mask Display: plot([-0.1, 1.05, NaN, -0.1, 1.05],[.01, .01, NaN, .99, .99]);
  stepDutyCycle : Assignment  IndexMode=Zero-based  IndexOptions=Index vector (port)  Indices=1  OutputSizes=1  mask(TL_Assignment){data={'insideiteratedsystem',logical(1),'omitinitializations',1,'output',{'variable','SAD/Vars/Steps/au16DutyCycle','inheritscaling',0},'date',738430.41691431717}}
      settings: CopyFcn=if exist('tl_reset_reviewflag') == 2, tl_reset_reviewflag(gcbh); end  DeleteFcn=if exist('delete_tlblock','file')==2,delete_tlblock(gcbh);end  NameChangeFcn=if exist('rename_tlblock','file')==2,rename_tlblock(gcbh);end  OpenFcn=if exist('tl_open_blockdlg','file')==2,tl_open_blockdlg(gcbh);else,open_system(gcbh,'parameter');end
      mask Help: eval(['if exist(''tl_online_help'',''file'') == 2, tl_online_help(''Topic'',''TL_Assignment''),else, web([''jar:file:///'',matlabroot,''/help/toolbox/simulink/help.jar!/slref/' lower(get_param(gcbh,'Blocktype')) '.html''], ''-helpbrowser''),end'])
      mask Display: plot([-0.1, 1.05, NaN, -0.1, 1.05],[.01, .01, NaN, .99, .99]);
  au8StepIdx : Outport
  au16DutyCycle : Outport  Port=2
  au16RawOrder : Outport  Port=3
  as16Slope : Outport  Port=4
  au16CurrentTime : Outport  Port=5
  ab8IsInfinite : Outport  Port=6
  ab8IsRamp : Outport  Port=7
  au16StepDuration : Outport  Port=8
  au8StepConsign : Outport  Port=9
  au8StepOrder : Outport  Port=10
  au8ExecutedStep : Outport  Port=11
  ab8IsStepTerminated : Outport  Port=12
  au8ExecutedProfile : Outport  Port=13
  as32Integral : Outport  Port=14
  wires:
  u8LoopIdx/1 -> [loopIdx]
  u8ExecutedProfile/1 -> Assignment1/2
  [loopIdx] -> Assignment1/3
  b8IsStepTerminated/1 -> IsStepFinished/2
  [loopIdx] -> IsStepFinished/3
  u8ExecutedStep/1 -> ExecutedStep/2
  [loopIdx] -> ExecutedStep/3
  u8StepOrderType/1 -> StepOrder/2
  [loopIdx] -> StepOrder/3
  u8StepConsign/1 -> StepConsign/2
  [loopIdx] -> StepConsign/3
  u16StepDuration/1 -> StepDuration/2
  [loopIdx] -> StepDuration/3
  b8StepIsRamp/1 -> IsRamp/2
  [loopIdx] -> IsRamp/3
  b8StepIsPID/1 -> IsPID/2
  [loopIdx] -> IsPID/3
  CurrentTime/1 -> au16CurrentTime/1
  u16CurrentTime/1 -> CurrentTime/2
  [loopIdx] -> CurrentTime/3
  StepIdx/1 -> au8StepIdx/1
  u8StepIdx/1 -> StepIdx/2
  [loopIdx] -> StepIdx/3
  stepDutyCycle/1 -> au16DutyCycle/1
  u16DutyCycle/1 -> stepDutyCycle/2
  [loopIdx] -> stepDutyCycle/3
  rawOrder/1 -> au16RawOrder/1
  u16RawOrder/1 -> rawOrder/2
  [loopIdx] -> rawOrder/3
  slope/1 -> as16Slope/1
  s16Slope/1 -> slope/2
  [loopIdx] -> slope/3
  IsPID/1 -> ab8IsInfinite/1
  IsRamp/1 -> ab8IsRamp/1
  StepDuration/1 -> au16StepDuration/1
  IsStepFinished/1 -> ab8IsStepTerminated/1
  Assignment1/1 -> au8ExecutedProfile/1
  Constant/1 -> IsRamp/1
  Constant1/1 -> IsPID/1
  Constant2/1 -> CurrentTime/1
  Constant3/1 -> StepIdx/1
  Constant4/1 -> stepDutyCycle/1
  Constant5/1 -> rawOrder/1
  Constant6/1 -> slope/1
  Constant7/1 -> StepDuration/1
  Constant8/1 -> StepConsign/1
  Constant9/1 -> StepOrder/1
  Constant10/1 -> ExecutedStep/1
  Constant11/1 -> IsStepFinished/1
  Constant12/1 -> Assignment1/1
  Integral/1 -> as32Integral/1
  s32Integral/1 -> Integral/2
  [loopIdx] -> Integral/3
  Constant13/1 -> Integral/1
  StepConsign/1 -> au8StepConsign/1
  StepOrder/1 -> au8StepOrder/1
  ExecutedStep/1 -> au8ExecutedStep/1

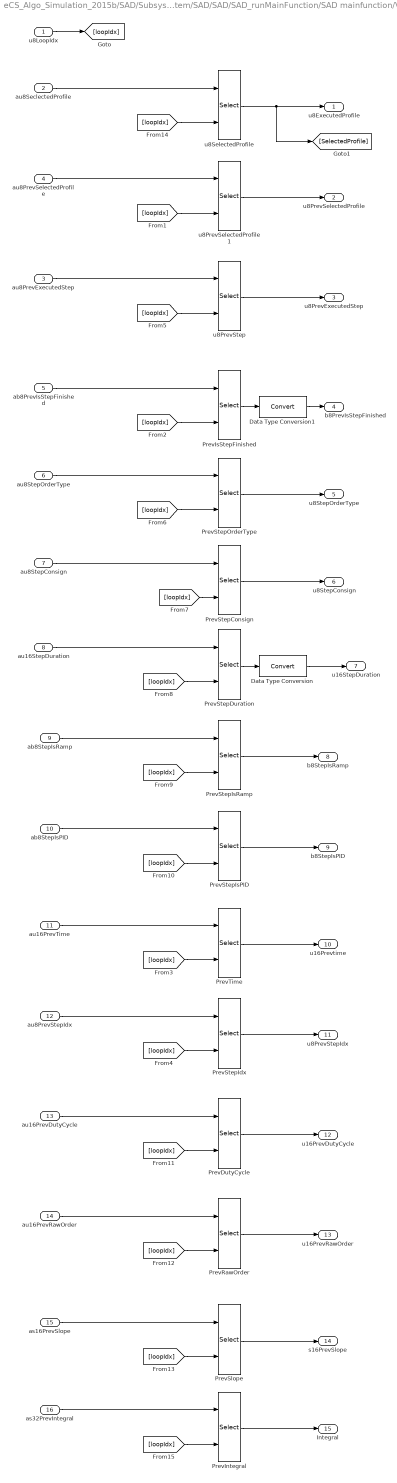
== system eCS_Algo_Simulation_2015b/SAD/Subsystem/SAD/SAD/SAD_runMainFunction/SAD mainfunction/VectorToScalar ==
  u8LoopIdx : Inport
  au8SeclectedProfile : Inport  Port=2
  au8PrevExecutedStep : Inport  Port=3
  au8PrevSelectedProfile : Inport  Port=4
  ab8PrevIsStepFinished : Inport  Port=5
  au8StepOrderType : Inport  Port=6
  au8StepConsign : Inport  Port=7
  au16StepDuration : Inport  Port=8
  ab8StepIsRamp : Inport  Port=9
  ab8StepIsPID : Inport  Port=10
  au16PrevTime : Inport  Port=11
  au8PrevStepIdx : Inport  Port=12
  au16PrevDutyCycle : Inport  Port=13
  au16PrevRawOrder : Inport  Port=14
  as16PrevSlope : Inport  Port=15
  as32PrevIntegral : Inport  Port=16
  Data Type Conversion : DataTypeConversion
  Data Type Conversion1 : DataTypeConversion
  PrevDutyCycle : Selector  IndexMode=Zero-based  IndexOptions=Index vector (port)  Indices=[1 3]  OutputSizes=1
  PrevIntegral : Selector  IndexMode=Zero-based  IndexOptions=Index vector (port)  Indices=[1 3]  OutputSizes=1
  PrevIsStepFinished : Selector  IndexMode=Zero-based  IndexOptions=Index vector (port)  Indices=[1 3]  OutputSizes=1
  PrevRawOrder : Selector  IndexMode=Zero-based  IndexOptions=Index vector (port)  Indices=[1 3]  OutputSizes=1
  PrevSlope : Selector  IndexMode=Zero-based  IndexOptions=Index vector (port)  Indices=[1 3]  OutputSizes=1
  PrevStepConsign : Selector  IndexMode=Zero-based  IndexOptions=Index vector (port)  Indices=[1 3]  OutputSizes=1
  PrevStepDuration : Selector  IndexMode=Zero-based  IndexOptions=Index vector (port)  Indices=[1 3]  OutputSizes=1
  PrevStepIdx : Selector  IndexMode=Zero-based  IndexOptions=Index vector (port)  Indices=[1 3]  OutputSizes=1
  PrevStepIsPID : Selector  IndexMode=Zero-based  IndexOptions=Index vector (port)  Indices=[1 3]  OutputSizes=1
  PrevStepIsRamp : Selector  IndexMode=Zero-based  IndexOptions=Index vector (port)  Indices=[1 3]  OutputSizes=1
  PrevStepOrderType : Selector  IndexMode=Zero-based  IndexOptions=Index vector (port)  Indices=[1 3]  OutputSizes=1
  PrevTime : Selector  IndexMode=Zero-based  IndexOptions=Index vector (port)  Indices=[1 3]  OutputSizes=1
  u8PrevSelectedProfile1 : Selector  IndexMode=Zero-based  IndexOptions=Index vector (port)  Indices=[1 3]  OutputSizes=1
  u8PrevStep : Selector  IndexMode=Zero-based  IndexOptions=Index vector (port)  Indices=[1 3]  OutputSizes=1
  u8SelectedProfile : Selector  IndexMode=Zero-based  IndexOptions=Index vector (port)  Indices=[1 3]  OutputSizes=1
  u8ExecutedProfile : Outport
  u8PrevSelectedProfile : Outport  Port=2
  u8PrevExecutedStep : Outport  Port=3
  b8PrevIsStepFinished : Outport  Port=4
  u8StepOrderType : Outport  Port=5
  u8StepConsign : Outport  Port=6
  u16StepDuration : Outport  Port=7
  b8StepIsRamp : Outport  Port=8
  b8StepIsPID : Outport  Port=9
  u16Prevtime : Outport  Port=10
  u8PrevStepIdx : Outport  Port=11
  u16PrevDutyCycle : Outport  Port=12
  u16PrevRawOrder : Outport  Port=13
  s16PrevSlope : Outport  Port=14
  Integral : Outport  Port=15
  wires:
  u8PrevStep/1 -> u8PrevExecutedStep/1
  [loopIdx] -> u8PrevStep/2
  au8PrevExecutedStep/1 -> u8PrevStep/1
  [loopIdx] -> u8SelectedProfile/2
  au8SeclectedProfile/1 -> u8SelectedProfile/1
  u8SelectedProfile/1 -> [SelectedProfile], u8ExecutedProfile/1
  u8LoopIdx/1 -> [loopIdx]
  [loopIdx] -> u8PrevSelectedProfile1/2
  au8PrevSelectedProfile/1 -> u8PrevSelectedProfile1/1
  u8PrevSelectedProfile1/1 -> u8PrevSelectedProfile/1
  ab8PrevIsStepFinished/1 -> PrevIsStepFinished/1
  [loopIdx] -> PrevIsStepFinished/2
  PrevIsStepFinished/1 -> Data Type Conversion1/1
  PrevStepIsPID/1 -> b8StepIsPID/1
  PrevStepIsRamp/1 -> b8StepIsRamp/1
  PrevStepDuration/1 -> Data Type Conversion/1
  PrevStepConsign/1 -> u8StepConsign/1
  PrevStepOrderType/1 -> u8StepOrderType/1
  au8StepOrderType/1 -> PrevStepOrderType/1
  [loopIdx] -> PrevStepOrderType/2
  au8StepConsign/1 -> PrevStepConsign/1
  [loopIdx] -> PrevStepConsign/2
  au16StepDuration/1 -> PrevStepDuration/1
  [loopIdx] -> PrevStepDuration/2
  ab8StepIsRamp/1 -> PrevStepIsRamp/1
  [loopIdx] -> PrevStepIsRamp/2
  ab8StepIsPID/1 -> PrevStepIsPID/1
  [loopIdx] -> PrevStepIsPID/2
  Data Type Conversion/1 -> u16StepDuration/1
  Data Type Conversion1/1 -> b8PrevIsStepFinished/1
  PrevTime/1 -> u16Prevtime/1
  au16PrevTime/1 -> PrevTime/1
  [loopIdx] -> PrevTime/2
  PrevStepIdx/1 -> u8PrevStepIdx/1
  au8PrevStepIdx/1 -> PrevStepIdx/1
  [loopIdx] -> PrevStepIdx/2
  PrevDutyCycle/1 -> u16PrevDutyCycle/1
  au16PrevDutyCycle/1 -> PrevDutyCycle/1
  [loopIdx] -> PrevDutyCycle/2
  au16PrevRawOrder/1 -> PrevRawOrder/1
  [loopIdx] -> PrevRawOrder/2
  PrevRawOrder/1 -> u16PrevRawOrder/1
  as16PrevSlope/1 -> PrevSlope/1
  [loopIdx] -> PrevSlope/2
  PrevSlope/1 -> s16PrevSlope/1
  as32PrevIntegral/1 -> PrevIntegral/1
  [loopIdx] -> PrevIntegral/2
  PrevIntegral/1 -> Integral/1
